simulink model "Rengen1"  (R2016a)
settings: Solver=VariableStepAuto  StartTime=0.0  StopTime=10.0  RelTol=1e-3
undefined symbols (not defined in the file): Ion, Lithium
libraries: powerlib x10, powerlib_meascontrol x5, electricdrivelib x1
settings Model: Creator=EBUKA  LastModifiedBy=EBUKA
settings GRTTargetCC: GeneratePreprocessorConditionals=Use local settings

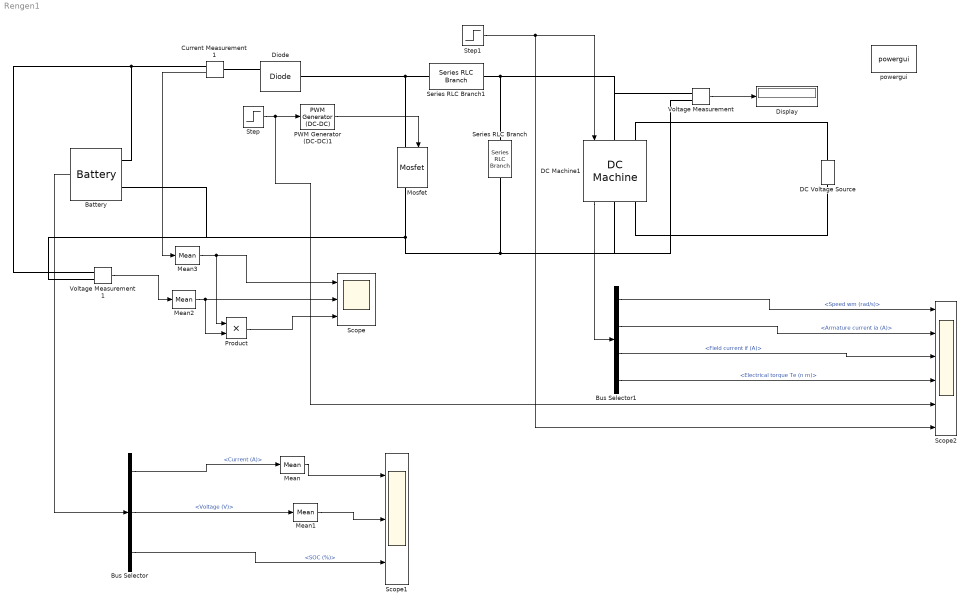
== system Rengen1 ==
  Battery : electricdrivelib/Extra Sources/Battery  BatType=Lithium-Ion  ShowTempParam=off  ThermalPreset=no  NomV=240  NomQ=15.5  SOC=50  Batt_Tr=30  PresetModel=on  MaxQ=15.5  MinV=180  FullV=279.3569  Dis_rate=6.7391  R=0.15484  Normal_OP=14.0174  expZone="[259.2926     0.7615217]"  current=[6.5 13 32.5]  Units=Time  Tci=20  NomT=25  T2=0  MaxQ2=2.208  FullV2=3.45  Normal_OP2=2.8  expZone2="[3.22        0.23]"  Rca=0.6  ti=1000  Dp=0
  Bus Selector : BusSelector  OutputSignals=Current (A),Voltage (V),SOC (%)
  Bus Selector1 : BusSelector  OutputSignals=Speed wm (rad/s),Armature current ia (A),Field current if (A),Electrical torque Te (n m)
  Current Measurement1 : powerlib/Measurements/Current Measurement  PhasorSimulation=off  OutputType=Complex  PSBequivalent=0
  DC Machine1 : powerlib/Machines/DC Machine  PresetModel=01: 5HP 240V 1750RPM Field:300V  MechanicalLoad=Torque TL  FieldType=Wound  ShowDetailedParameters=on  MeasurementBus=off  RLa=[2.581 0.028]  RLf=[281.3 156]  Laf=0.9483  MachineConstant=Torque constant (N.m/A)  Ke=1.8  Kt=1.8  J=0.02215  Bm=0.002953  Tf=0.5161  w0=1  Ifinit=1  TsPowergui=0  TsBlock=-1
  DC Voltage Source : powerlib/Electrical Sources/DC Voltage Source  Amplitude=300  Measurements=None
  Diode : powerlib/Power Electronics/Diode  Ron=0.001  Lon=0  Vf=0.8  IC=0  UseSnubber=off  Rs=500  Cs=250e-9  Measurements=on
  Display : Display
  Mean{,1..3} (4 alike) : powerlib_meascontrol/Measurements/Mean  Freq=60  Vinit=0  Ts=0
  Mosfet : powerlib/Power Electronics/Mosfet  Ron=0.1  Lon=0  Rd=0.01  Vfd=0  IC=0  Rs=1e5  Cs=inf  Measurements=on
  PWM Generator (DC-DC)1 : powerlib_meascontrol/Pulse & Signal Generators/PWM Generator (DC-DC)  Fsw=5000  Ts=0
  Product : Product
  Scope : Scope  NumInputPorts=3
  Scope1 : Scope  NumInputPorts=3
  Scope2 : Scope  NumInputPorts=6
  Series RLC Branch : powerlib/Elements/Series RLC Branch  LConnTagsString=__new0  RConnTagsString=__new0  BranchType=C  Resistance=1  Inductance=1e-3  SetiL0=off  InitialCurrent=0  Capacitance=150e-6  Setx0=off  InitialVoltage=0  Measurements=None
  Series RLC Branch1 : powerlib/Elements/Series RLC Branch  LConnTagsString=__new0  RConnTagsString=__new0  BranchType=L  Resistance=1  Inductance=5e-3  SetiL0=off  InitialCurrent=0  Capacitance=1e-6  Setx0=off  InitialVoltage=0  Measurements=None
  Step : Step  Time=3  Before=0.6  After=0.8  SampleTime=0
  Step1 : Step  Time=7  Before=-20  After=-5  SampleTime=0
  Voltage Measurement : powerlib/Measurements/Voltage Measurement  PhasorSimulation=off  OutputType=Complex  PSBequivalent=0
  Voltage Measurement1 : powerlib/Measurements/Voltage Measurement  PhasorSimulation=off  OutputType=Complex  PSBequivalent=0
  powergui : powerlib/powergui  Priority=1  SimulationMode=Continuous  SolverType=Tustin/Backward Euler (TBE)  SampleTime=50e-6  frequency=60  SPID=off  DisableSnubberDevices=off  DisableRonSwitches=off  DisableVfSwitches=off  SwTol=0  DisplayEquations=off  Interpol=off  ExternalGateDelay=off  methode=off  Ts=10  FunctionMessages=off  echomessages=off  HookPort=off  EnableUseOfTLC=off  x0status=blocks  frequencyindice=0  Pbase=100e6  ErrMax=1e-4  Iterations=50  UnitsV=kV  UnitsW=MW  buscounter=0  RestoreLinks=warning  ResistiveCurrentMeasurement=off  Frange=[0:2:500]  Ylog=off  Xlog=on  ShowGrid=off  save=off  variable=ZData  structure=0  ZoomFFT=off  StartTime=0.0  cycles=1  DisplayStyle=1  fundamental=60  FreqAxis=off  MaxFrequency=1000  frequencyindicesteady=1  RmsSteady=1  display=off
  wires:
  DC Machine1/1 -> Bus Selector1/1
  Voltage Measurement/1 -> Display/1
  Bus Selector1/1 -> Scope2/1  "<Speed wm (rad/s)>"
  Bus Selector1/2 -> Scope2/2  "<Armature current ia (A)>"
  Bus Selector1/3 -> Scope2/3  "<Field current if (A)>"
  Step1/1 -> DC Machine1/1, Scope2/6
  Bus Selector1/4 -> Scope2/4  "<Electrical torque Te (n m)>"
  PWM Generator (DC-DC)1/1 -> Mosfet/1
  Step/1 -> PWM Generator (DC-DC)1/1, Scope2/5
  Mean/1 -> Scope1/1
  Mean1/1 -> Scope1/2
  Battery/1 -> Bus Selector/1
  Bus Selector/2 -> Mean1/1  "<Voltage (V)>"
  Product/1 -> Scope/3
  Mean3/1 -> Product/1, Scope/1
  Mean2/1 -> Product/2, Scope/2
  Voltage Measurement1/1 -> Mean2/1
  Current Measurement1/1 -> Mean3/1
  Bus Selector/1 -> Mean/1  "<Current (A)>"
  Bus Selector/3 -> Scope1/3  "<SOC (%)>"
  connections:
  Series RLC Branch1/LConn1 -- Diode/LConn1 -- Mosfet/LConn1
  Series RLC Branch1/RConn1 -- DC Machine1/LConn1 -- Voltage Measurement/LConn1 -- Series RLC Branch/LConn1
  DC Machine1/RConn1 -- Voltage Measurement/LConn2 -- Battery/LConn2 -- Voltage Measurement1/LConn2 -- Mosfet/RConn1 -- Series RLC Branch/RConn1
  DC Voltage Source/LConn1 -- DC Machine1/RConn2
  DC Machine1/LConn2 -- DC Voltage Source/RConn1
  Current Measurement1/LConn1 -- Diode/RConn1
  Current Measurement1/RConn1 -- Battery/LConn1 -- Voltage Measurement1/LConn1
